simulink model "autoMBD_example_defaultConfig"  (R2020b)
settings: Solver=FixedStepAuto  StartTime=0.0  StopTime=10.0  FixedStep=0.001  RelTol=1e-3
settings Model: Creator=k  LastModifiedBy=k
settings OptimizationCC: DefaultParameterBehavior=Inlined  EnhancedBackFolding=on  PassReuseOutputArgsAs=Individual arguments  ZeroExternalMemoryAtStartup=off  ZeroInternalMemoryAtStartup=off  OptimizeBlockOrder=speed  DifferentSizesBufferReuse=on  OptimizationCustomize=off  EfficientTunableParamExpr=on
settings DebuggingCC: ParameterTunabilityLossMsg=error
settings SFSimCC: MATLABDynamicMemAlloc=off
settings RTWCC: Description=Embedded Coder  SystemTargetFile=ert.tlc  GenCodeOnly=on  TemplateMakefile=ert_default_tmf
settings CodeAppCC: ForceParamTrailComments=on  IgnoreCustomStorageClasses=off  OperatorAnnotations=on  SimulinkDataObjDesc=on  SFDataObjDesc=on  InsertBlockDesc=on
settings ERTTargetCC: TargetLangStandard=C99 (ISO)  GenerateSampleERTMain=on  InlinedParameterPlacement=NonHierarchical  ERTCustomFileTemplate=example_file_process.tlc

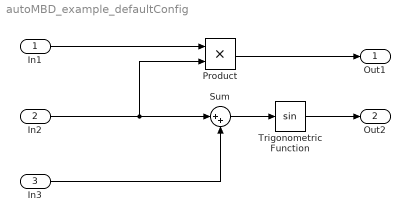
== system autoMBD_example_defaultConfig ==
  In1 : Inport
  In2 : Inport  Port=2
  In3 : Inport  Port=3
  Product : Product
  Sum : Sum  Inputs=|++
  Trigonometric Function : Trigonometry
  Out1 : Outport
  Out2 : Outport  Port=2
  wires:
  In1/1 -> Product/1
  In2/1 -> Product/2, Sum/1
  In3/1 -> Sum/2
  Product/1 -> Out1/1
  Sum/1 -> Trigonometric Function/1
  Trigonometric Function/1 -> Out2/1
